simulink model "Droop_control_conditioning_untouched"  (R2024b)
settings: Solver=ode4  StartTime=0.0  StopTime=2  FixedStep=Ts  RelTol=1e-3
InitFcn:
  | %% Droop Control
  | m1=0.5e-5; % f-P droop gain
  | n1=5e-3;   % Q-V droop gain
  | fn=50;  % nominal frequency
  | Vn=325;  % nominal voltage
  | wc=2*pi*5;  % cut off frequency of low pass filter used in droop control
  | 
  | %% Voltage Controller
  | 
  | kpv=1;  % voltage controller proportional gain
  | kiv=189; % voltage controller integral gain
  | F=0.75;  % Feedforeward gain
  | Ilim1=40; % voltage controller limit
  | Ilim2=-40; % voltage controller limit
  | 
  | %% Current controller
  | 
  | kpi=10.47*2;  % current controller proportional gain
  | kii=4188.8*4; % current controller integral gain
  | Vlim1=500; % current controller limit
  | Vlim2=500; % current controller limit
  | 
  | %% System parameter
  | Lf=1.6e-3; % filter inductance
  | Cf=50e-6;  % filter capacitance
  | Rc=0.03;   % Coupling resistance
  | Lc=0.35e-3;% Coupling inducatnace
  | fs=10e3;    % switching frequency
  | Ts=10e-7;    % sample time
  | Vin=1000;   % DC voltage or input of inverter
  | Tsample=20*Ts;
  | ts=0.04; % black start time in step block used in Q-V droop controller and at PWM
  | 
  | %% Line parameters
  | R1=0.23; % line resistance
  | L1=3.1e-4;  %line inducatance
libraries: spsSeriesRLCBranchLib x9, slpidlib x8, spsThreePhaseSeriesRLCBranchLib x7, spsabctodq0Lib x6, spsGroundLib x5, spsThreePhaseVIMeasurementLib x5, spsDCVoltageSourceLib x2, spsPowerdq0InstantaneousLib x2, spsPWMGenerator2LevelLib x2, spsUniversalBridgeLib x2, spsdq0toabcLib x2, dspstat3 x1
(part 1 of 2)
settings Model: SimulationMode=accelerator  Creator=praki  LastModifiedBy=praki
settings DataIOCC: SaveFormat=StructureWithTime
settings RTWCC: GPUComputeCapability=3.5

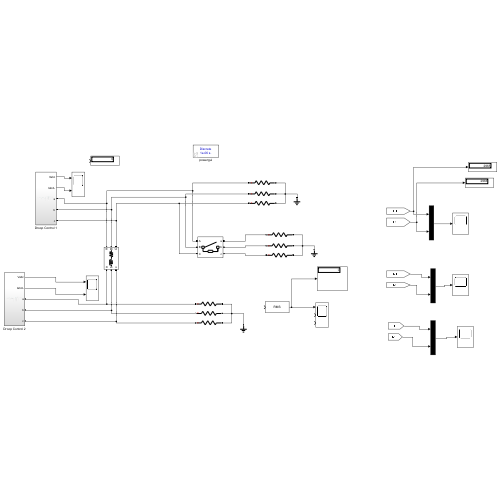
[thumbnail: Simulink's stored preview of the top-level diagram]
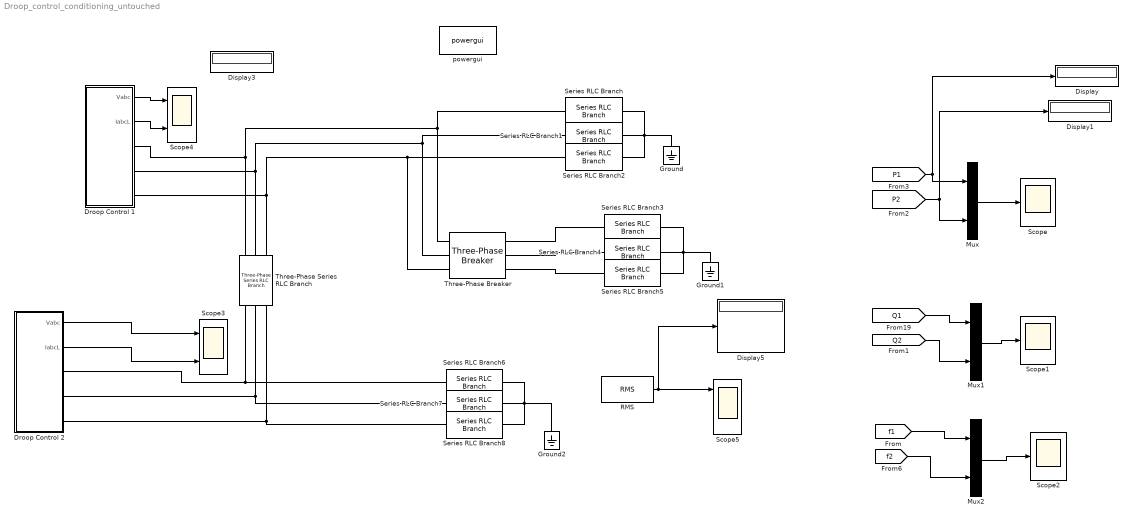
== system Droop_control_conditioning_untouched ==
  Display{,1,3,5} (4 alike) : Display
  Droop Control 1 : Subsystem
  Droop Control 2 : Subsystem
  Ground : spsGroundLib/Ground  LConnTagsString=a
  Ground1 : spsGroundLib/Ground  LConnTagsString=a
  Ground2 : spsGroundLib/Ground  LConnTagsString=a
  Mux : Mux  Inputs=2
  Mux1 : Mux  Inputs=2
  Mux2 : Mux  Inputs=2
  RMS : dspstat3/RMS  run=off  directionMode=Each column  dimension=1  InputProcessing=Columns as channels (frame based)  reset_popup=None
  Scope : Scope
  Scope1 : Scope
  Scope2 : Scope
  Scope3 : Scope  NumInputPorts=2
  Scope4 : Scope  NumInputPorts=2
  Scope5 : Scope  NumInputPorts=3
  Series RLC Branch : spsSeriesRLCBranchLib/Series RLC Branch  LConnTagsString=__new0  RConnTagsString=__new0  BranchType=R  Resistance=32  Inductance=1e-3  SetiL0=off  InitialCurrent=0  Capacitance=1e-6  Setx0=off  InitialVoltage=0  Measurements=None
  Series RLC Branch1 : spsSeriesRLCBranchLib/Series RLC Branch  LConnTagsString=__new0  RConnTagsString=__new0  BranchType=R  Resistance=32  Inductance=1e-3  SetiL0=off  InitialCurrent=0  Capacitance=1e-6  Setx0=off  InitialVoltage=0  Measurements=None
  Series RLC Branch2 : spsSeriesRLCBranchLib/Series RLC Branch  LConnTagsString=__new0  RConnTagsString=__new0  BranchType=R  Resistance=32  Inductance=1e-3  SetiL0=off  InitialCurrent=0  Capacitance=1e-6  Setx0=off  InitialVoltage=0  Measurements=None
  Series RLC Branch{3..8} (6 alike) : spsSeriesRLCBranchLib/Series RLC Branch  LConnTagsString=__new0  RConnTagsString=__new0  BranchType=R  Resistance=160  Inductance=1e-3  SetiL0=off  InitialCurrent=0  Capacitance=1e-6  Setx0=off  InitialVoltage=0  Measurements=None
  Three-Phase Series RLC Branch : spsThreePhaseSeriesRLCBranchLib/Three-Phase Series RLC Branch  LConnTagsString=A|B|C  RConnTagsString=A|B|C  BranchType=RL  Resistance=R1  Inductance=L1  Capacitance=1e-6  Measurements=None
  Three-Phase Breaker : spsThreePhaseBreakerLib/Three-Phase Breaker  InitialState=open  SwitchA=on  SwitchB=on  SwitchC=on  SwitchTimes=[1]  External=off  BreakerResistance=0.01  SnubberResistance=1e6  SnubberCapacitance=inf  Measurements=None
  powergui : sps_lib/powergui  Priority=1  SimulationMode=Discrete  SampleTime=Ts  frequency=60  Iterations=50  frequencyindice=0  Pbase=100e6  ErrMax=1e-4  UnitsV=kV  UnitsW=MW  buscounter=0  FunctionMessages=off  echomessages=off  EnableUseOfTLC=off  CurrentSourceSwitches=off  DisableSnubberDevices=off  DisableRonSwitches=off  DisableVfSwitches=off  DisplayEquations=off  AutomaticDiscreteSolvers=off  SolverType=Tustin/Backward Euler (TBE)  Interpol=off  ExternalGateDelay=off  methode=off  Ts=100  x0status=blocks  SPID=on  SwTol=0  HookPort=off  NonlinearTolerance=1e-4  nMaxIteration=100  ContinueOnMaxIteration=off  RestoreLinks=warning  ResistiveCurrentMeasurement=off  Frange=[0:2:500]  Ylog=off  Xlog=on  ShowGrid=off  save=off  variable=ZData  structure=0  ZoomFFT=off  StartTime=0.0  cycles=1  DisplayStyle=1  fundamental=60  FreqAxis=off  MaxFrequency=1000  frequencyindicesteady=1  RmsSteady=1  display=off
  wires:
  [P1] -> Display/1, Mux/1
  [f2] -> Mux2/2
  [P2] -> Display1/1, Mux/2
  Mux/1 -> Scope/1
  Mux2/1 -> Scope2/1
  [f1] -> Mux2/1
  Mux1/1 -> Scope1/1
  [Q1] -> Mux1/1
  [Q2] -> Mux1/2
  RMS/1 -> Display5/1, Scope5/1
  Droop Control 1/1(Vabc) -> Scope4/1
  Droop Control 1/2(IabcL) -> Scope4/2
  Droop Control 2/1(Vabc) -> Scope3/1
  Droop Control 2/2(IabcL) -> Scope3/2
  connections:
  Three-Phase Breaker/LConn2 -- Series RLC Branch1/LConn1 -- Three-Phase Series RLC Branch/LConn2 -- Droop Control 1/RConn2
  Three-Phase Breaker/LConn3 -- Series RLC Branch2/LConn1 -- Three-Phase Series RLC Branch/LConn3 -- Droop Control 1/RConn3
  Three-Phase Breaker/LConn1 -- Series RLC Branch/LConn1 -- Three-Phase Series RLC Branch/LConn1 -- Droop Control 1/RConn1
  Droop Control 2/RConn1 -- Three-Phase Series RLC Branch/RConn1 -- Series RLC Branch6/LConn1
  Droop Control 2/RConn2 -- Series RLC Branch7/LConn1 -- Three-Phase Series RLC Branch/RConn2
  Droop Control 2/RConn3 -- Series RLC Branch8/LConn1 -- Three-Phase Series RLC Branch/RConn3
  Series RLC Branch/RConn1 -- Series RLC Branch1/RConn1 -- Ground/LConn1 -- Series RLC Branch2/RConn1
  Series RLC Branch4/RConn1 -- Series RLC Branch5/RConn1 -- Ground1/LConn1 -- Series RLC Branch3/RConn1
  Series RLC Branch3/LConn1 -- Three-Phase Breaker/RConn1
  Three-Phase Breaker/RConn2 -- Series RLC Branch4/LConn1
  Three-Phase Breaker/RConn3 -- Series RLC Branch5/LConn1
  Series RLC Branch8/RConn1 -- Ground2/LConn1 -- Series RLC Branch7/RConn1 -- Series RLC Branch6/RConn1

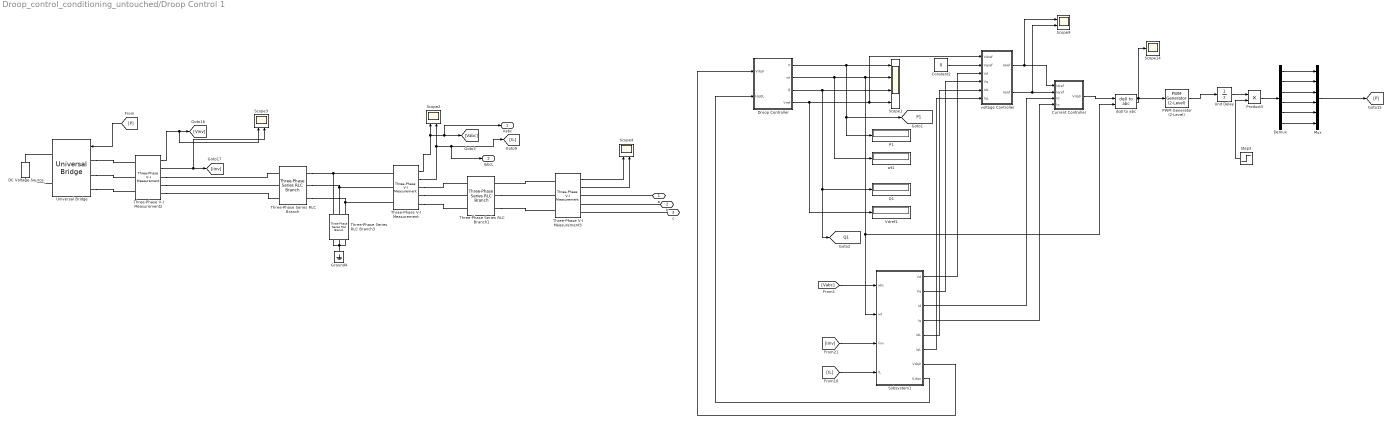
== system Droop_control_conditioning_untouched/Droop Control 1 ==
  Constant2 : Constant  Value=0
  Current Controller : Subsystem
  DC Voltage Source : spsDCVoltageSourceLib/DC Voltage Source  Amplitude=Vin  Measurements=None
  Demux : Demux  Outputs=6
  Droop Controller : Subsystem
  Ground4 : spsGroundLib/Ground  LConnTagsString=a
  Mux : Mux  Inputs=6
  P1 : Display
  PWM Generator (2-Level) : spsPWMGenerator2LevelLib/PWM Generator (2-Level)  ModulatorType=Three-phase bridge (6 pulses)  ModulatorMode=Unsynchronized  Fc=fs  Pc=90  nF=27  MinMax="[ -1  1 ]"  SamplingTechnique=Natural  ModulatingSignals=off  m=0.8  Freq=60  Phase=0  Ts=Ts  ShowCarrierOutport=off
  Product3 : Product  Inputs=**
  Q1 : Display
  Scope1 : Scope  NumInputPorts=4
  Scope14 : Scope
  Scope{2..4,9} (4 alike) : Scope  NumInputPorts=2
  Step3 : Step  Time=ts  SampleTime=0
  Subsystem1 : Subsystem
  Three-Phase Series RLC Branch : spsThreePhaseSeriesRLCBranchLib/Three-Phase Series RLC Branch  LConnTagsString=A|B|C  RConnTagsString=A|B|C  BranchType=RL  Resistance=0.2  Inductance=Lf  Capacitance=1e-6  Measurements=None
  Three-Phase Series RLC Branch1 : spsThreePhaseSeriesRLCBranchLib/Three-Phase Series RLC Branch  LConnTagsString=A|B|C  RConnTagsString=A|B|C  BranchType=RL  Resistance=Rc  Inductance=Lc  Capacitance=1e-6  Measurements=None
  Three-Phase Series RLC Branch3 : spsThreePhaseSeriesRLCBranchLib/Three-Phase Series RLC Branch  LConnTagsString=A|B|C  RConnTagsString=A|B|C  BranchType=C  Resistance=0.2  Inductance=50e-6  Capacitance=Cf  Measurements=None
  Three-Phase V-I Measurement : spsThreePhaseVIMeasurementLib/Three-Phase V-I Measurement  VoltageMeasurement=phase-to-ground  SetLabelV=off  LabelV=Vabc  Vpu=off  VpuLL=off  CurrentMeasurement=yes  SetLabelI=off  LabelI=Iload  Ipu=off  Pbase=100e6  Vbase=500e3  OutputType=Complex  PhasorSimulation=off  PSBequivalent=0
  Three-Phase V-I Measurement2 : spsThreePhaseVIMeasurementLib/Three-Phase V-I Measurement  VoltageMeasurement=phase-to-ground  SetLabelV=off  LabelV=Vabc  Vpu=off  VpuLL=off  CurrentMeasurement=yes  SetLabelI=off  LabelI=Iload  Ipu=off  Pbase=100e6  Vbase=500e3  OutputType=Complex  PhasorSimulation=off  PSBequivalent=0
  Three-Phase V-I Measurement3 : spsThreePhaseVIMeasurementLib/Three-Phase V-I Measurement  VoltageMeasurement=phase-to-ground  SetLabelV=off  LabelV=Vabc  Vpu=off  VpuLL=off  CurrentMeasurement=yes  SetLabelI=off  LabelI=Iload  Ipu=off  Pbase=100e6  Vbase=500e3  OutputType=Complex  PhasorSimulation=off  PSBequivalent=0
  Unit Delay : UnitDelay  SampleTime=Ts  HasFrameUpgradeWarning=on
  Universal Bridge : spsUniversalBridgeLib/Universal Bridge  Arms=3  SnubberResistance=1e5  SnubberCapacitance=inf  Device=IGBT / Diodes  Ron=1e-3  Lon=0  ForwardVoltages="[  0  0  ]"  ForwardVoltage=0  GTOparameters=[ 10e-6 , 20e-6 ]  IGBTparameters=[ 1e-6 , 2e-6 ]  Measurements=None  Measurements_2=None  converterType=Rectifier
  Vdref1 : Display
  dq0 to abc : spsdq0toabcLib/dq0 to abc  Alignment=90 degrees behind phase A axis
  voltage Controller : Subsystem
  wt1 : Display
  a : PMIOPort  Side=Right
  b : PMIOPort  Port=2  Side=Right
  c : PMIOPort  Port=3  Side=Right
  Vabc : Outport
  IabcL : Outport  Port=2
  tag scope: P1=global, Q1=global
  wires:
  Constant2/1 -> voltage Controller/2(Vqref)
  Three-Phase V-I Measurement/2 -> IabcL/1, [IL], Scope2/2
  Subsystem1/2(Vq) -> voltage Controller/4(Vq)
  Droop Controller/1(P) -> P1/1, [P1], Scope1/1
  Droop Controller/2(wt) -> wt1/1, Scope1/2, Subsystem1/2(wt), dq0 to abc/2
  Three-Phase V-I Measurement2/1 -> [Vinv], Scope3/1
  Three-Phase V-I Measurement/1 -> Vabc/1, [Vabc], Scope2/1
  [Iinv] -> Subsystem1/3(Iinv)
  Droop Controller/4(Vref) -> Vdref1/1, voltage Controller/1(Vdref), Scope1/4
  Droop Controller/3(Q) -> Q1/1, [Q1], Scope1/3
  dq0 to abc/1 -> PWM Generator (2-Level)/1, Scope14/1
  Subsystem1/3(Id) -> Current Controller/3(Id)
  [P] -> Universal Bridge/1
  Subsystem1/5(IdL) -> voltage Controller/5(IdL)
  Step3/1 -> Product3/2
  Subsystem1/8(ILdqo) -> Droop Controller/2(Idq0L)
  voltage Controller/1(Idref) -> Current Controller/1(Idref), Scope9/1
  Subsystem1/4(Iq) -> Current Controller/4(Iq)
  Unit Delay/1 -> Product3/1
  [Vabc] -> Subsystem1/1(abc)
  Subsystem1/6(IqL) -> voltage Controller/6(IqL)
  Subsystem1/7(Vdq0) -> Droop Controller/1(Vdq0)
  Three-Phase V-I Measurement2/2 -> Scope3/2, [Iinv]
  Current Controller/1(Vdq0) -> dq0 to abc/1
  Subsystem1/1(Vd) -> voltage Controller/3(Vd)
  [IL] -> Subsystem1/4(IL)
  voltage Controller/2(Iqref) -> Scope9/2, Current Controller/2(Iqref)
  Three-Phase V-I Measurement3/1 -> Scope4/1
  Three-Phase V-I Measurement3/2 -> Scope4/2
  PWM Generator (2-Level)/1 -> Unit Delay/1
  Demux/1 -> Mux/1
  Demux/2 -> Mux/2
  Demux/3 -> Mux/3
  Demux/4 -> Mux/4
  Demux/6 -> Mux/6
  Demux/5 -> Mux/5
  Product3/1 -> Demux/1
  Mux/1 -> [P]
  connections:
  DC Voltage Source/RConn1 -- Universal Bridge/RConn1
  Three-Phase V-I Measurement2/RConn1 -- Three-Phase Series RLC Branch/LConn1
  Three-Phase Series RLC Branch3/RConn2 -- Ground4/LConn1 -- Three-Phase Series RLC Branch3/RConn1 -- Three-Phase Series RLC Branch3/RConn3
  Three-Phase V-I Measurement2/RConn2 -- Three-Phase Series RLC Branch/LConn2
  Universal Bridge/LConn3 -- Three-Phase V-I Measurement2/LConn3
  Three-Phase Series RLC Branch/RConn3 -- Three-Phase V-I Measurement/LConn3 -- Three-Phase Series RLC Branch3/LConn3
  Three-Phase Series RLC Branch/RConn2 -- Three-Phase V-I Measurement/LConn2 -- Three-Phase Series RLC Branch3/LConn2
  Universal Bridge/LConn1 -- Three-Phase V-I Measurement2/LConn1
  Three-Phase Series RLC Branch/RConn1 -- Three-Phase V-I Measurement/LConn1 -- Three-Phase Series RLC Branch3/LConn1
  Universal Bridge/RConn2 -- DC Voltage Source/LConn1
  Three-Phase V-I Measurement2/RConn3 -- Three-Phase Series RLC Branch/LConn3
  Universal Bridge/LConn2 -- Three-Phase V-I Measurement2/LConn2
  Three-Phase V-I Measurement/RConn1 -- Three-Phase Series RLC Branch1/LConn1
  Three-Phase V-I Measurement/RConn2 -- Three-Phase Series RLC Branch1/LConn2
  Three-Phase V-I Measurement/RConn3 -- Three-Phase Series RLC Branch1/LConn3
  Three-Phase V-I Measurement3/LConn1 -- Three-Phase Series RLC Branch1/RConn1
  Three-Phase Series RLC Branch1/RConn2 -- Three-Phase V-I Measurement3/LConn2
  Three-Phase Series RLC Branch1/RConn3 -- Three-Phase V-I Measurement3/LConn3
  a/RConn1 -- Three-Phase V-I Measurement3/RConn1
  b/RConn1 -- Three-Phase V-I Measurement3/RConn2
  c/RConn1 -- Three-Phase V-I Measurement3/RConn3

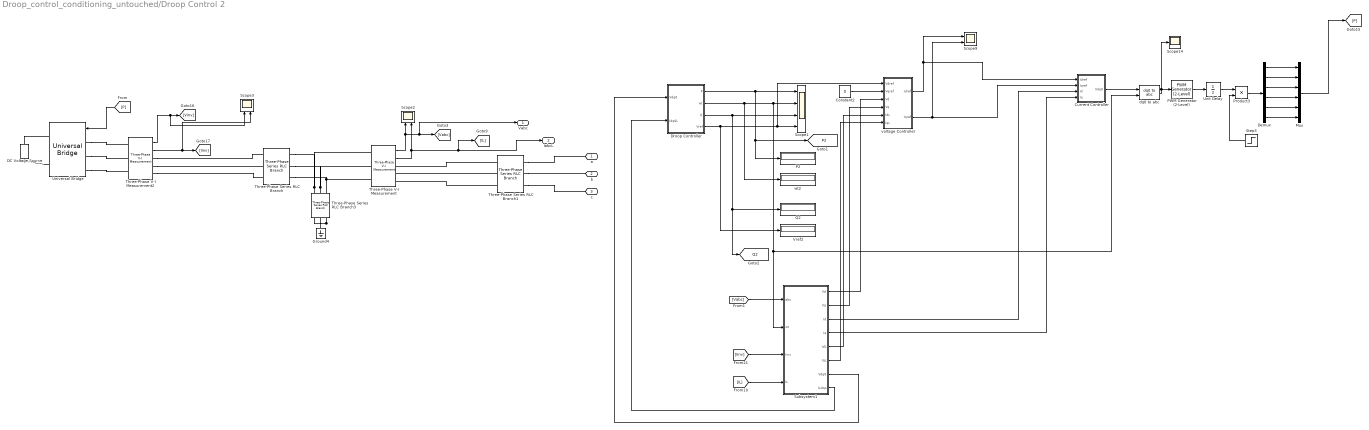
== system Droop_control_conditioning_untouched/Droop Control 2 ==
  Constant2 : Constant  Value=0
  Current Controller : Subsystem
  DC Voltage Source : spsDCVoltageSourceLib/DC Voltage Source  Amplitude=Vin  Measurements=None
  Demux : Demux  Outputs=6
  Droop Controller : Subsystem
  Ground4 : spsGroundLib/Ground  LConnTagsString=a
  Mux : Mux  Inputs=6
  P2 : Display
  PWM Generator (2-Level) : spsPWMGenerator2LevelLib/PWM Generator (2-Level)  ModulatorType=Three-phase bridge (6 pulses)  ModulatorMode=Unsynchronized  Fc=fs  Pc=90  nF=27  MinMax="[ -1  1 ]"  SamplingTechnique=Natural  ModulatingSignals=off  m=0.8  Freq=60  Phase=0  Ts=Ts  ShowCarrierOutport=off
  Product3 : Product  Inputs=**
  Q2 : Display
  Scope1 : Scope  NumInputPorts=4
  Scope14 : Scope
  Scope2 : Scope  NumInputPorts=2
  Scope3 : Scope  NumInputPorts=2
  Scope9 : Scope  NumInputPorts=2
  Step3 : Step  Time=ts  SampleTime=0
  Subsystem1 : Subsystem
  Three-Phase Series RLC Branch : spsThreePhaseSeriesRLCBranchLib/Three-Phase Series RLC Branch  LConnTagsString=A|B|C  RConnTagsString=A|B|C  BranchType=RL  Resistance=0.2  Inductance=Lf  Capacitance=1e-6  Measurements=None
  Three-Phase Series RLC Branch1 : spsThreePhaseSeriesRLCBranchLib/Three-Phase Series RLC Branch  LConnTagsString=A|B|C  RConnTagsString=A|B|C  BranchType=RL  Resistance=Rc  Inductance=Lc  Capacitance=1e-6  Measurements=None
  Three-Phase Series RLC Branch3 : spsThreePhaseSeriesRLCBranchLib/Three-Phase Series RLC Branch  LConnTagsString=A|B|C  RConnTagsString=A|B|C  BranchType=C  Resistance=0.2  Inductance=50e-6  Capacitance=Cf  Measurements=None
  Three-Phase V-I Measurement : spsThreePhaseVIMeasurementLib/Three-Phase V-I Measurement  VoltageMeasurement=phase-to-ground  SetLabelV=off  LabelV=Vabc  Vpu=off  VpuLL=off  CurrentMeasurement=yes  SetLabelI=off  LabelI=Iload  Ipu=off  Pbase=100e6  Vbase=500e3  OutputType=Complex  PhasorSimulation=off  PSBequivalent=0
  Three-Phase V-I Measurement2 : spsThreePhaseVIMeasurementLib/Three-Phase V-I Measurement  VoltageMeasurement=phase-to-ground  SetLabelV=off  LabelV=Vabc  Vpu=off  VpuLL=off  CurrentMeasurement=yes  SetLabelI=off  LabelI=Iload  Ipu=off  Pbase=100e6  Vbase=500e3  OutputType=Complex  PhasorSimulation=off  PSBequivalent=0
  Unit Delay : UnitDelay  SampleTime=Ts  HasFrameUpgradeWarning=on
  Universal Bridge : spsUniversalBridgeLib/Universal Bridge  Arms=3  SnubberResistance=1e5  SnubberCapacitance=inf  Device=IGBT / Diodes  Ron=1e-3  Lon=0  ForwardVoltages="[  0  0  ]"  ForwardVoltage=0  GTOparameters=[ 10e-6 , 20e-6 ]  IGBTparameters=[ 1e-6 , 2e-6 ]  Measurements=None  Measurements_2=None  converterType=Rectifier
  Vref2 : Display
  dq0 to abc : spsdq0toabcLib/dq0 to abc  Alignment=90 degrees behind phase A axis
  voltage Controller : Subsystem
  wt2 : Display
  a : PMIOPort  Side=Right
  b : PMIOPort  Port=2  Side=Right
  c : PMIOPort  Port=3  Side=Right
  Vabc : Outport
  IabcL : Outport  Port=2
  tag scope: P2=global, Q2=global
  wires:
  [IL] -> Subsystem1/4(IL)
  Subsystem1/1(Vd) -> voltage Controller/3(Vd)
  Current Controller/1(Vdq0) -> dq0 to abc/1
  Three-Phase V-I Measurement2/2 -> [Iinv], Scope3/2
  Subsystem1/7(Vdq0) -> Droop Controller/1(Vdq0)
  Subsystem1/6(IqL) -> voltage Controller/6(IqL)
  [Vabc] -> Subsystem1/1(abc)
  Unit Delay/1 -> Product3/1
  Subsystem1/4(Iq) -> Current Controller/4(Iq)
  voltage Controller/1(Idref) -> Current Controller/1(Idref), Scope9/1
  Subsystem1/8(ILdqo) -> Droop Controller/2(Idq0L)
  Step3/1 -> Product3/2
  Subsystem1/5(IdL) -> voltage Controller/5(IdL)
  [P] -> Universal Bridge/1
  Subsystem1/3(Id) -> Current Controller/3(Id)
  dq0 to abc/1 -> Scope14/1, PWM Generator (2-Level)/1
  Droop Controller/3(Q) -> Scope1/3, [Q2], Q2/1
  Droop Controller/4(Vref) -> Scope1/4, voltage Controller/1(Vdref), Vref2/1
  [Iinv] -> Subsystem1/3(Iinv)
  Three-Phase V-I Measurement/1 -> Scope2/1, Vabc/1, [Vabc]
  Three-Phase V-I Measurement2/1 -> Scope3/1, [Vinv]
  Droop Controller/2(wt) -> dq0 to abc/2, Subsystem1/2(wt), Scope1/2, wt2/1
  Droop Controller/1(P) -> Scope1/1, [P2], P2/1
  Subsystem1/2(Vq) -> voltage Controller/4(Vq)
  Three-Phase V-I Measurement/2 -> Scope2/2, IabcL/1, [IL]
  Constant2/1 -> voltage Controller/2(Vqref)
  voltage Controller/2(Iqref) -> Scope9/2, Current Controller/2(Iqref)
  PWM Generator (2-Level)/1 -> Unit Delay/1
  Mux/1 -> [P]
  Demux/5 -> Mux/5
  Product3/1 -> Demux/1
  Demux/3 -> Mux/3
  Demux/2 -> Mux/2
  Demux/1 -> Mux/1
  Demux/4 -> Mux/4
  Demux/6 -> Mux/6
  connections:
  Universal Bridge/LConn2 -- Three-Phase V-I Measurement2/LConn2
  Three-Phase V-I Measurement2/RConn3 -- Three-Phase Series RLC Branch/LConn3
  Universal Bridge/RConn2 -- DC Voltage Source/LConn1
  Three-Phase Series RLC Branch3/LConn1 -- Three-Phase Series RLC Branch/RConn1 -- Three-Phase V-I Measurement/LConn1
  Universal Bridge/LConn1 -- Three-Phase V-I Measurement2/LConn1
  Three-Phase Series RLC Branch3/LConn2 -- Three-Phase Series RLC Branch/RConn2 -- Three-Phase V-I Measurement/LConn2
  Three-Phase Series RLC Branch/RConn3 -- Three-Phase V-I Measurement/LConn3 -- Three-Phase Series RLC Branch3/LConn3
  Universal Bridge/LConn3 -- Three-Phase V-I Measurement2/LConn3
  Three-Phase V-I Measurement2/RConn2 -- Three-Phase Series RLC Branch/LConn2
  Three-Phase Series RLC Branch3/RConn3 -- Three-Phase Series RLC Branch3/RConn1 -- Three-Phase Series RLC Branch3/RConn2 -- Ground4/LConn1
  Three-Phase V-I Measurement2/RConn1 -- Three-Phase Series RLC Branch/LConn1
  DC Voltage Source/RConn1 -- Universal Bridge/RConn1
  Three-Phase Series RLC Branch1/LConn1 -- Three-Phase V-I Measurement/RConn1
  Three-Phase Series RLC Branch1/LConn2 -- Three-Phase V-I Measurement/RConn2
  Three-Phase Series RLC Branch1/LConn3 -- Three-Phase V-I Measurement/RConn3
  Three-Phase Series RLC Branch1/RConn1 -- a/RConn1
  Three-Phase Series RLC Branch1/RConn2 -- b/RConn1
  Three-Phase Series RLC Branch1/RConn3 -- c/RConn1

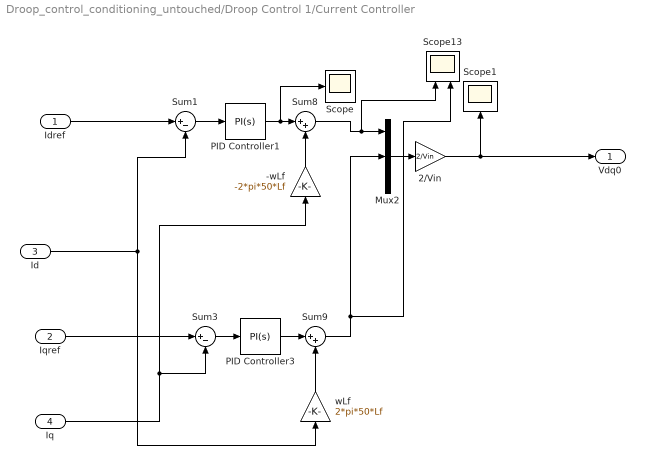
== system Droop_control_conditioning_untouched/Droop Control 1/Current Controller ==
  Idref : Inport
  Iqref : Inport  Port=2
  Id : Inport  Port=3
  Iq : Inport  Port=4
  -wLf : Gain  Gain=-2*pi*50*Lf
  2/Vin : Gain  Gain=2/Vin
  Mux2 : Mux  Inputs=3
  PID Controller1 : slpidlib/PID Controller  Controller=PI  Form=Parallel  TimeDomain=Continuous-time  UseExternalTs=off  SampleTime=Tsample  IntegratorMethod=Forward Euler  FilterMethod=Forward Euler  ControllerParametersSource=internal  P=kpi  I=kii  UseKiTs=off  D=0  UseExternalDerivativeSource=off  N=100  UseFilter=on  TunerSelectOption=Transfer Function Based (PID Tuner App)  InitialConditionSource=internal  InitialConditionForIntegrator=0  InitialConditionForFilter=0  DifferentiatorICPrevScaledInput=0  ExternalReset=none  TrackingMode=off  Kt=1  LimitOutput=off  SatLimitsSource=internal  UpperSaturationLimit=Vlim1  LowerSaturationLimit=Vlim2  LinearizeAsGain=on  AntiWindupMode=none  Kb=1  LimitIntegrator=off  UpperIntegratorSaturationLimit=inf  LowerIntegratorSaturationLimit=-inf  POutMin=[]  POutMax=[]  IOutMin=[]  IOutMax=[]  DOutMin=[]  DOutMax=[]  NOutMin=[]  NOutMax=[]  SumOutMin=[]  SumOutMax=[]  SaturationOutMin=[]  SaturationOutMax=[]  PParamMin=[]  PParamMax=[]  IParamMin=[]  IParamMax=[]  DParamMin=[]  DParamMax=[]  NParamMin=[]  NParamMax=[]  KbParamMin=[]  KbParamMax=[]  KtParamMin=[]  KtParamMax=[]  KbOutMin=[]  KbOutMax=[]  KtOutMin=[]  KtOutMax=[]  IntegratorOutMin=[]  IntegratorOutMax=[]  FilterOutMin=[]  FilterOutMax=[]  SumI1OutMin=[]  SumI1OutMax=[]  SumI2OutMin=[]  SumI2OutMax=[]  SumI3OutMin=[]  SumI3OutMax=[]  SumI4OutMin=[]  SumI4OutMax=[]  SumDOutMin=[]  SumDOutMax=[]  DifferentiatorOutMin=[]  DifferentiatorOutMax=[]  FilterDiffOutCoefMin=[]  FilterDiffOutCoefMax=[]  ReciprocalOutMin=[]  ReciprocalOutMax=[]  SumDenOutMin=[]  SumDenOutMax=[]  SumNumOutMin=[]  SumNumOutMax=[]  DivideOutMin=[]  DivideOutMax=[]  UdiffTsProdOutMin=[]  UdiffTsProdOutMax=[]  NTsProdOutMin=[]  NTsProdOutMax=[]  UintegralTsProdOutMin=[]  UintegralTsProdOutMax=[]  UngainTsProdOutMin=[]  UngainTsProdOutMax=[]  ClampingZeroOutDataTypeStr=Inherit: Inherit via back propagation  ClampingZeroOutMin=[]  ClampingZeroOutMax=[]  FilterDenConstantOutDataTypeStr=Inherit: Inherit via back propagation  FilterDenConstantOutMin=[]  FilterDenConstantOutMax=[]  PCopyOutDataTypeStr=Inherit: Inherit via back propagation  PCopyOutMin=[]  PCopyOutMax=[]  NCopyOutDataTypeStr=Inherit: Inherit via back propagation  NCopyOutMin=[]  NCopyOutMax=[]  IntegratorContinuousStateAttributes=''  IntegratorStateMustResolveToSignalObject=off  IntegratorRTWStateStorageClass=Auto  FilterContinuousStateAttributes=''  FilterStateMustResolveToSignalObject=off  FilterRTWStateStorageClass=Auto  ParallelPVariant=InternalParameters  IdealPVariant=Disabled  IVariant=InternalParameters  DVariant=Disabled  IntegratorVariant=Continuous  SatVariant=Disabled  AWVariant=Passthrough  PCopyVariant=Disabled  TRVariant=Disabled  FdbkBlocksVariant=Forward  IdealPFdbkVariant=Disabled  SatFdbkVariant=Disabled  DerivativeFilterVariant=Disabled  NVariant=Disabled  NCopyVariant=Disabled_SignalSpec  FilterICVariant=Disabled  IntegratorICVariant=InternalICs  ExternalResetVariant=Disabled  TRSumVariant=Passthrough  SumFdbkVariant=Disabled  SumVariant=Sum_PI  TsampFilterVariant=InternalTs  TsampNgainVariant=Passthrough  TsampIntegralVariant=Disabled_SignalSpec  ExternalSaturationOutDataTypeStr=Inherit: Same as second input  DerivativeSourceVariant=Disabled  PreIntVariant=InternalPreInt
  PID Controller3 : slpidlib/PID Controller  Controller=PI  Form=Parallel  TimeDomain=Continuous-time  UseExternalTs=off  SampleTime=Tsample  IntegratorMethod=Forward Euler  FilterMethod=Forward Euler  ControllerParametersSource=internal  P=kpi  I=kii  UseKiTs=off  D=0  UseExternalDerivativeSource=off  N=100  UseFilter=on  TunerSelectOption=Transfer Function Based (PID Tuner App)  InitialConditionSource=internal  InitialConditionForIntegrator=0  InitialConditionForFilter=0  DifferentiatorICPrevScaledInput=0  ExternalReset=none  TrackingMode=off  Kt=1  LimitOutput=off  SatLimitsSource=internal  UpperSaturationLimit=Vlim1  LowerSaturationLimit=Vlim2  LinearizeAsGain=on  AntiWindupMode=none  Kb=1  LimitIntegrator=off  UpperIntegratorSaturationLimit=inf  LowerIntegratorSaturationLimit=-inf  POutMin=[]  POutMax=[]  IOutMin=[]  IOutMax=[]  DOutMin=[]  DOutMax=[]  NOutMin=[]  NOutMax=[]  SumOutMin=[]  SumOutMax=[]  SaturationOutMin=[]  SaturationOutMax=[]  PParamMin=[]  PParamMax=[]  IParamMin=[]  IParamMax=[]  DParamMin=[]  DParamMax=[]  NParamMin=[]  NParamMax=[]  KbParamMin=[]  KbParamMax=[]  KtParamMin=[]  KtParamMax=[]  KbOutMin=[]  KbOutMax=[]  KtOutMin=[]  KtOutMax=[]  IntegratorOutMin=[]  IntegratorOutMax=[]  FilterOutMin=[]  FilterOutMax=[]  SumI1OutMin=[]  SumI1OutMax=[]  SumI2OutMin=[]  SumI2OutMax=[]  SumI3OutMin=[]  SumI3OutMax=[]  SumI4OutMin=[]  SumI4OutMax=[]  SumDOutMin=[]  SumDOutMax=[]  DifferentiatorOutMin=[]  DifferentiatorOutMax=[]  FilterDiffOutCoefMin=[]  FilterDiffOutCoefMax=[]  ReciprocalOutMin=[]  ReciprocalOutMax=[]  SumDenOutMin=[]  SumDenOutMax=[]  SumNumOutMin=[]  SumNumOutMax=[]  DivideOutMin=[]  DivideOutMax=[]  UdiffTsProdOutMin=[]  UdiffTsProdOutMax=[]  NTsProdOutMin=[]  NTsProdOutMax=[]  UintegralTsProdOutMin=[]  UintegralTsProdOutMax=[]  UngainTsProdOutMin=[]  UngainTsProdOutMax=[]  ClampingZeroOutDataTypeStr=Inherit: Inherit via back propagation  ClampingZeroOutMin=[]  ClampingZeroOutMax=[]  FilterDenConstantOutDataTypeStr=Inherit: Inherit via back propagation  FilterDenConstantOutMin=[]  FilterDenConstantOutMax=[]  PCopyOutDataTypeStr=Inherit: Inherit via back propagation  PCopyOutMin=[]  PCopyOutMax=[]  NCopyOutDataTypeStr=Inherit: Inherit via back propagation  NCopyOutMin=[]  NCopyOutMax=[]  IntegratorContinuousStateAttributes=''  IntegratorStateMustResolveToSignalObject=off  IntegratorRTWStateStorageClass=Auto  FilterContinuousStateAttributes=''  FilterStateMustResolveToSignalObject=off  FilterRTWStateStorageClass=Auto  ParallelPVariant=InternalParameters  IdealPVariant=Disabled  IVariant=InternalParameters  DVariant=Disabled  IntegratorVariant=Continuous  SatVariant=Disabled  AWVariant=Passthrough  PCopyVariant=Disabled  TRVariant=Disabled  FdbkBlocksVariant=Forward  IdealPFdbkVariant=Disabled  SatFdbkVariant=Disabled  DerivativeFilterVariant=Disabled  NVariant=Disabled  NCopyVariant=Disabled_SignalSpec  FilterICVariant=Disabled  IntegratorICVariant=InternalICs  ExternalResetVariant=Disabled  TRSumVariant=Passthrough  SumFdbkVariant=Disabled  SumVariant=Sum_PI  TsampFilterVariant=InternalTs  TsampNgainVariant=Passthrough  TsampIntegralVariant=Disabled_SignalSpec  ExternalSaturationOutDataTypeStr=Inherit: Same as second input  DerivativeSourceVariant=Disabled  PreIntVariant=InternalPreInt
  Scope : Scope
  Scope1 : Scope
  Scope13 : Scope  NumInputPorts=2
  Sum1 : Sum  Inputs=|+-
  Sum3 : Sum  Inputs=|+-
  Sum8 : Sum  Inputs=|++
  Sum9 : Sum  Inputs=|++
  wLf : Gain  Gain=2*pi*50*Lf
  Vdq0 : Outport
  wires:
  Sum9/1 -> Scope13/2, Mux2/2
  wLf/1 -> Sum9/2
  2/Vin/1 -> Vdq0/1, Scope1/1
  Id/1 -> Sum1/2, wLf/1
  Iq/1 -> -wLf/1, Sum3/2
  Sum1/1 -> PID Controller1/1
  PID Controller3/1 -> Sum9/1
  Sum8/1 -> Scope13/1, Mux2/1
  Sum3/1 -> PID Controller3/1
  PID Controller1/1 -> Scope/1, Sum8/1
  Mux2/1 -> 2/Vin/1
  Idref/1 -> Sum1/1
  -wLf/1 -> Sum8/2
  Iqref/1 -> Sum3/1

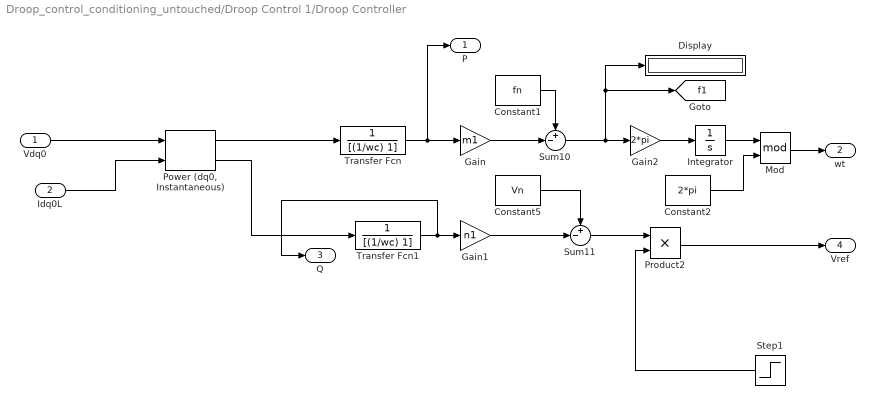
== system Droop_control_conditioning_untouched/Droop Control 1/Droop Controller ==
  Vdq0 : Inport
  Idq0L : Inport  Port=2
  Constant1 : Constant  Value=fn
  Constant2 : Constant  Value=2*pi
  Constant5 : Constant  Value=Vn
  Display : Display
  Gain : Gain  Gain=m1
  Gain1 : Gain  Gain=n1
  Gain2 : Gain  Gain=2*pi
  Integrator : Integrator
  Mod : Math  Operator=mod
  "Power (dq0, Instantaneous)" : spsPowerdq0InstantaneousLib/Power (dq0, Instantaneous)
      settings: LibrarySourceBlock=|
      | sps_lib/Sensors and Measurements/Power
      | (dq0, Instantaneous)
  Product2 : Product  Inputs=**
  Step1 : Step  Time=ts  SampleTime=0
  Sum10 : Sum  Inputs=+-|
  Sum11 : Sum  Inputs=+-|
  Transfer Fcn : TransferFcn  Numerator=[0 1]  Denominator=[(1/wc) 1]
  Transfer Fcn1 : TransferFcn  Numerator=[0 1]  Denominator=[(1/wc) 1]
  P : Outport
  wt : Outport  Port=2
  Q : Outport  Port=3
  Vref : Outport  Port=4
  tag scope: f1=global
  wires:
  "Power (dq0, Instantaneous)"/2 -> Transfer Fcn1/1
  "Power (dq0, Instantaneous)"/1 -> Transfer Fcn/1
  Constant1/1 -> Sum10/1
  Constant5/1 -> Sum11/1
  Gain1/1 -> Sum11/2
  Gain/1 -> Sum10/2
  Transfer Fcn/1 -> P/1, Gain/1
  Transfer Fcn1/1 -> Q/1, Gain1/1
  Integrator/1 -> Mod/1
  Mod/1 -> wt/1
  Constant2/1 -> Mod/2
  Vdq0/1 -> "Power (dq0, Instantaneous)"/1
  Idq0L/1 -> "Power (dq0, Instantaneous)"/2
  Gain2/1 -> Integrator/1
  Sum10/1 -> Gain2/1, [f1], Display/1
  Step1/1 -> Product2/2
  Product2/1 -> Vref/1
  Sum11/1 -> Product2/1

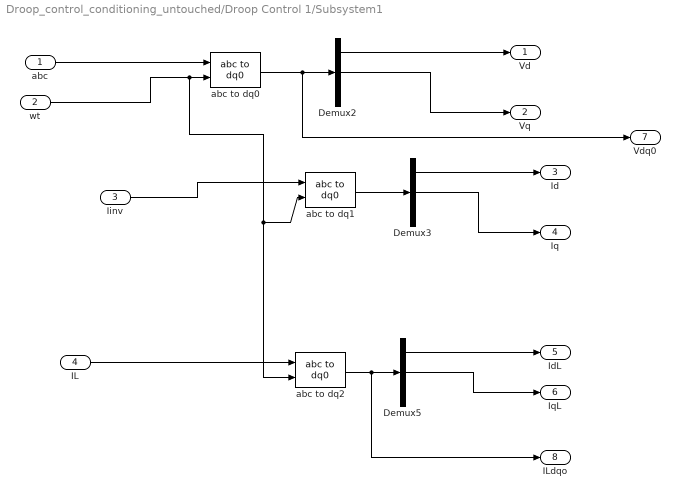
== system Droop_control_conditioning_untouched/Droop Control 1/Subsystem1 ==
  abc : Inport
  wt : Inport  Port=2
  Iinv : Inport  Port=3
  IL : Inport  Port=4
  Demux2 : Demux  Outputs=3
  Demux3 : Demux  Outputs=3
  Demux5 : Demux  Outputs=3
  abc to dq0 : spsabctodq0Lib/abc to dq0  Alignment=90 degrees behind phase A axis
  abc to dq1 : spsabctodq0Lib/abc to dq0  Alignment=90 degrees behind phase A axis
  abc to dq2 : spsabctodq0Lib/abc to dq0  Alignment=90 degrees behind phase A axis
  Vd : Outport
  Vq : Outport  Port=2
  Id : Outport  Port=3
  Iq : Outport  Port=4
  IdL : Outport  Port=5
  IqL : Outport  Port=6
  Vdq0 : Outport  Port=7
  ILdqo : Outport  Port=8
  wires:
  abc to dq0/1 -> Vdq0/1, Demux2/1
  abc to dq2/1 -> ILdqo/1, Demux5/1
  abc to dq1/1 -> Demux3/1
  wt/1 -> abc to dq2/2, abc to dq1/2, abc to dq0/2
  Demux2/2 -> Vq/1
  Iinv/1 -> abc to dq1/1
  Demux3/1 -> Id/1
  Demux2/1 -> Vd/1
  Demux5/1 -> IdL/1
  Demux5/2 -> IqL/1
  abc/1 -> abc to dq0/1
  Demux3/2 -> Iq/1
  IL/1 -> abc to dq2/1

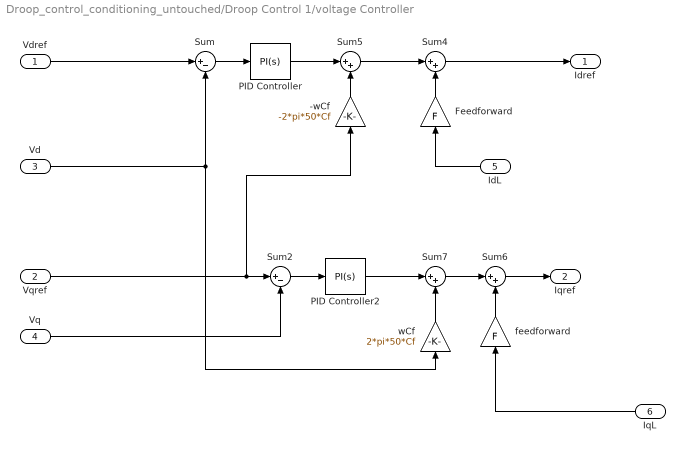
== system Droop_control_conditioning_untouched/Droop Control 1/voltage Controller ==
  Vdref : Inport
  Vqref : Inport  Port=2
  Vd : Inport  Port=3
  Vq : Inport  Port=4
  IdL : Inport  Port=5
  IqL : Inport  Port=6
  -wCf : Gain  Gain=-2*pi*50*Cf
  Feedforward : Gain  Gain=F
  PID Controller : slpidlib/PID Controller  Controller=PI  Form=Parallel  TimeDomain=Continuous-time  UseExternalTs=off  SampleTime=Tsample  IntegratorMethod=Forward Euler  FilterMethod=Forward Euler  ControllerParametersSource=internal  P=kpv  I=kiv  UseKiTs=off  D=0  UseExternalDerivativeSource=off  N=100  UseFilter=on  TunerSelectOption=Transfer Function Based (PID Tuner App)  InitialConditionSource=internal  InitialConditionForIntegrator=0  InitialConditionForFilter=0  DifferentiatorICPrevScaledInput=0  ExternalReset=none  TrackingMode=off  Kt=1  LimitOutput=off  SatLimitsSource=internal  UpperSaturationLimit=Ilim1  LowerSaturationLimit=Ilim2  LinearizeAsGain=off  AntiWindupMode=none  Kb=1  LimitIntegrator=off  UpperIntegratorSaturationLimit=inf  LowerIntegratorSaturationLimit=-inf  POutMin=[]  POutMax=[]  IOutMin=[]  IOutMax=[]  DOutMin=[]  DOutMax=[]  NOutMin=[]  NOutMax=[]  SumOutMin=[]  SumOutMax=[]  SaturationOutMin=[]  SaturationOutMax=[]  PParamMin=[]  PParamMax=[]  IParamMin=[]  IParamMax=[]  DParamMin=[]  DParamMax=[]  NParamMin=[]  NParamMax=[]  KbParamMin=[]  KbParamMax=[]  KtParamMin=[]  KtParamMax=[]  KbOutMin=[]  KbOutMax=[]  KtOutMin=[]  KtOutMax=[]  IntegratorOutMin=[]  IntegratorOutMax=[]  FilterOutMin=[]  FilterOutMax=[]  SumI1OutMin=[]  SumI1OutMax=[]  SumI2OutMin=[]  SumI2OutMax=[]  SumI3OutMin=[]  SumI3OutMax=[]  SumI4OutMin=[]  SumI4OutMax=[]  SumDOutMin=[]  SumDOutMax=[]  DifferentiatorOutMin=[]  DifferentiatorOutMax=[]  FilterDiffOutCoefMin=[]  FilterDiffOutCoefMax=[]  ReciprocalOutMin=[]  ReciprocalOutMax=[]  SumDenOutMin=[]  SumDenOutMax=[]  SumNumOutMin=[]  SumNumOutMax=[]  DivideOutMin=[]  DivideOutMax=[]  UdiffTsProdOutMin=[]  UdiffTsProdOutMax=[]  NTsProdOutMin=[]  NTsProdOutMax=[]  UintegralTsProdOutMin=[]  UintegralTsProdOutMax=[]  UngainTsProdOutMin=[]  UngainTsProdOutMax=[]  ClampingZeroOutDataTypeStr=Inherit: Inherit via back propagation  ClampingZeroOutMin=[]  ClampingZeroOutMax=[]  FilterDenConstantOutDataTypeStr=Inherit: Inherit via back propagation  FilterDenConstantOutMin=[]  FilterDenConstantOutMax=[]  PCopyOutDataTypeStr=Inherit: Inherit via back propagation  PCopyOutMin=[]  PCopyOutMax=[]  NCopyOutDataTypeStr=Inherit: Inherit via back propagation  NCopyOutMin=[]  NCopyOutMax=[]  IntegratorContinuousStateAttributes=''  IntegratorStateMustResolveToSignalObject=off  IntegratorRTWStateStorageClass=Auto  FilterContinuousStateAttributes=''  FilterStateMustResolveToSignalObject=off  FilterRTWStateStorageClass=Auto  ParallelPVariant=InternalParameters  IdealPVariant=Disabled  IVariant=InternalParameters  DVariant=Disabled  IntegratorVariant=Continuous  SatVariant=Disabled  AWVariant=Passthrough  PCopyVariant=Disabled  TRVariant=Disabled  FdbkBlocksVariant=Forward  IdealPFdbkVariant=Disabled  SatFdbkVariant=Disabled  DerivativeFilterVariant=Disabled  NVariant=Disabled  NCopyVariant=Disabled_SignalSpec  FilterICVariant=Disabled  IntegratorICVariant=InternalICs  ExternalResetVariant=Disabled  TRSumVariant=Passthrough  SumFdbkVariant=Disabled  SumVariant=Sum_PI  TsampFilterVariant=InternalTs  TsampNgainVariant=Passthrough  TsampIntegralVariant=Disabled_SignalSpec  ExternalSaturationOutDataTypeStr=Inherit: Same as second input  DerivativeSourceVariant=Disabled  PreIntVariant=InternalPreInt
  PID Controller2 : slpidlib/PID Controller  Controller=PI  Form=Parallel  TimeDomain=Continuous-time  UseExternalTs=off  SampleTime=Tsample  IntegratorMethod=Forward Euler  FilterMethod=Forward Euler  ControllerParametersSource=internal  P=kpv  I=kiv  UseKiTs=off  D=0  UseExternalDerivativeSource=off  N=100  UseFilter=on  TunerSelectOption=Transfer Function Based (PID Tuner App)  InitialConditionSource=internal  InitialConditionForIntegrator=0  InitialConditionForFilter=0  DifferentiatorICPrevScaledInput=0  ExternalReset=none  TrackingMode=off  Kt=1  LimitOutput=off  SatLimitsSource=internal  UpperSaturationLimit=Ilim1  LowerSaturationLimit=Ilim2  LinearizeAsGain=off  AntiWindupMode=none  Kb=1  LimitIntegrator=off  UpperIntegratorSaturationLimit=inf  LowerIntegratorSaturationLimit=-inf  POutMin=[]  POutMax=[]  IOutMin=[]  IOutMax=[]  DOutMin=[]  DOutMax=[]  NOutMin=[]  NOutMax=[]  SumOutMin=[]  SumOutMax=[]  SaturationOutMin=[]  SaturationOutMax=[]  PParamMin=[]  PParamMax=[]  IParamMin=[]  IParamMax=[]  DParamMin=[]  DParamMax=[]  NParamMin=[]  NParamMax=[]  KbParamMin=[]  KbParamMax=[]  KtParamMin=[]  KtParamMax=[]  KbOutMin=[]  KbOutMax=[]  KtOutMin=[]  KtOutMax=[]  IntegratorOutMin=[]  IntegratorOutMax=[]  FilterOutMin=[]  FilterOutMax=[]  SumI1OutMin=[]  SumI1OutMax=[]  SumI2OutMin=[]  SumI2OutMax=[]  SumI3OutMin=[]  SumI3OutMax=[]  SumI4OutMin=[]  SumI4OutMax=[]  SumDOutMin=[]  SumDOutMax=[]  DifferentiatorOutMin=[]  DifferentiatorOutMax=[]  FilterDiffOutCoefMin=[]  FilterDiffOutCoefMax=[]  ReciprocalOutMin=[]  ReciprocalOutMax=[]  SumDenOutMin=[]  SumDenOutMax=[]  SumNumOutMin=[]  SumNumOutMax=[]  DivideOutMin=[]  DivideOutMax=[]  UdiffTsProdOutMin=[]  UdiffTsProdOutMax=[]  NTsProdOutMin=[]  NTsProdOutMax=[]  UintegralTsProdOutMin=[]  UintegralTsProdOutMax=[]  UngainTsProdOutMin=[]  UngainTsProdOutMax=[]  ClampingZeroOutDataTypeStr=Inherit: Inherit via back propagation  ClampingZeroOutMin=[]  ClampingZeroOutMax=[]  FilterDenConstantOutDataTypeStr=Inherit: Inherit via back propagation  FilterDenConstantOutMin=[]  FilterDenConstantOutMax=[]  PCopyOutDataTypeStr=Inherit: Inherit via back propagation  PCopyOutMin=[]  PCopyOutMax=[]  NCopyOutDataTypeStr=Inherit: Inherit via back propagation  NCopyOutMin=[]  NCopyOutMax=[]  IntegratorContinuousStateAttributes=''  IntegratorStateMustResolveToSignalObject=off  IntegratorRTWStateStorageClass=Auto  FilterContinuousStateAttributes=''  FilterStateMustResolveToSignalObject=off  FilterRTWStateStorageClass=Auto  ParallelPVariant=InternalParameters  IdealPVariant=Disabled  IVariant=InternalParameters  DVariant=Disabled  IntegratorVariant=Continuous  SatVariant=Disabled  AWVariant=Passthrough  PCopyVariant=Disabled  TRVariant=Disabled  FdbkBlocksVariant=Forward  IdealPFdbkVariant=Disabled  SatFdbkVariant=Disabled  DerivativeFilterVariant=Disabled  NVariant=Disabled  NCopyVariant=Disabled_SignalSpec  FilterICVariant=Disabled  IntegratorICVariant=InternalICs  ExternalResetVariant=Disabled  TRSumVariant=Passthrough  SumFdbkVariant=Disabled  SumVariant=Sum_PI  TsampFilterVariant=InternalTs  TsampNgainVariant=Passthrough  TsampIntegralVariant=Disabled_SignalSpec  ExternalSaturationOutDataTypeStr=Inherit: Same as second input  DerivativeSourceVariant=Disabled  PreIntVariant=InternalPreInt
  Sum : Sum  Inputs=|+-
  Sum2 : Sum  Inputs=|+-
  Sum{4..7} (4 alike) : Sum  Inputs=|++
  feedforward : Gain  Gain=F
  wCf : Gain  Gain=2*pi*50*Cf
  Idref : Outport
  Iqref : Outport  Port=2
  wires:
  Sum4/1 -> Idref/1
  Sum/1 -> PID Controller/1
  Sum5/1 -> Sum4/1
  feedforward/1 -> Sum6/2
  Sum7/1 -> Sum6/1
  IqL/1 -> feedforward/1
  Vd/1 -> Sum/2, wCf/1
  Vq/1 -> Sum2/2
  PID Controller2/1 -> Sum7/1
  Sum6/1 -> Iqref/1
  Feedforward/1 -> Sum4/2
  wCf/1 -> Sum7/2
  Sum2/1 -> PID Controller2/1
  -wCf/1 -> Sum5/2
  Vdref/1 -> Sum/1
  PID Controller/1 -> Sum5/1
  Vqref/1 -> -wCf/1, Sum2/1
  IdL/1 -> Feedforward/1

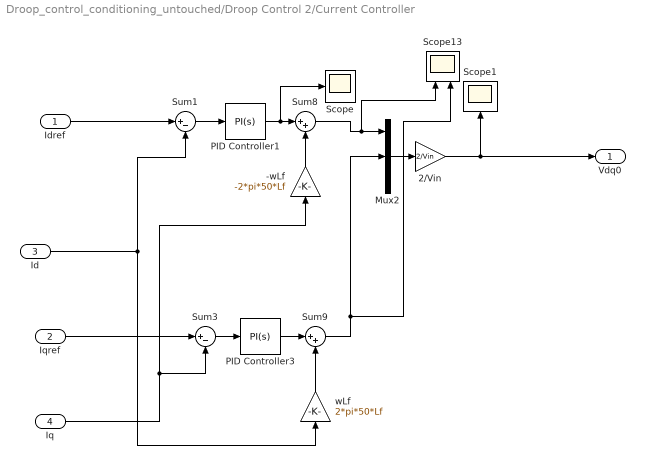
== system Droop_control_conditioning_untouched/Droop Control 2/Current Controller ==
  Idref : Inport
  Iqref : Inport  Port=2
  Id : Inport  Port=3
  Iq : Inport  Port=4
  -wLf : Gain  Gain=-2*pi*50*Lf
  2/Vin : Gain  Gain=2/Vin
  Mux2 : Mux  Inputs=3
  PID Controller1 : slpidlib/PID Controller  Controller=PI  Form=Parallel  TimeDomain=Continuous-time  UseExternalTs=off  SampleTime=Tsample  IntegratorMethod=Forward Euler  FilterMethod=Forward Euler  ControllerParametersSource=internal  P=kpi  I=kii  UseKiTs=off  D=0  UseExternalDerivativeSource=off  N=100  UseFilter=on  TunerSelectOption=Transfer Function Based (PID Tuner App)  InitialConditionSource=internal  InitialConditionForIntegrator=0  InitialConditionForFilter=0  DifferentiatorICPrevScaledInput=0  ExternalReset=none  TrackingMode=off  Kt=1  LimitOutput=off  SatLimitsSource=internal  UpperSaturationLimit=Ilim1  LowerSaturationLimit=Ilim2  LinearizeAsGain=on  AntiWindupMode=none  Kb=1  LimitIntegrator=off  UpperIntegratorSaturationLimit=inf  LowerIntegratorSaturationLimit=-inf  POutMin=[]  POutMax=[]  IOutMin=[]  IOutMax=[]  DOutMin=[]  DOutMax=[]  NOutMin=[]  NOutMax=[]  SumOutMin=[]  SumOutMax=[]  SaturationOutMin=[]  SaturationOutMax=[]  PParamMin=[]  PParamMax=[]  IParamMin=[]  IParamMax=[]  DParamMin=[]  DParamMax=[]  NParamMin=[]  NParamMax=[]  KbParamMin=[]  KbParamMax=[]  KtParamMin=[]  KtParamMax=[]  KbOutMin=[]  KbOutMax=[]  KtOutMin=[]  KtOutMax=[]  IntegratorOutMin=[]  IntegratorOutMax=[]  FilterOutMin=[]  FilterOutMax=[]  SumI1OutMin=[]  SumI1OutMax=[]  SumI2OutMin=[]  SumI2OutMax=[]  SumI3OutMin=[]  SumI3OutMax=[]  SumI4OutMin=[]  SumI4OutMax=[]  SumDOutMin=[]  SumDOutMax=[]  DifferentiatorOutMin=[]  DifferentiatorOutMax=[]  FilterDiffOutCoefMin=[]  FilterDiffOutCoefMax=[]  ReciprocalOutMin=[]  ReciprocalOutMax=[]  SumDenOutMin=[]  SumDenOutMax=[]  SumNumOutMin=[]  SumNumOutMax=[]  DivideOutMin=[]  DivideOutMax=[]  UdiffTsProdOutMin=[]  UdiffTsProdOutMax=[]  NTsProdOutMin=[]  NTsProdOutMax=[]  UintegralTsProdOutMin=[]  UintegralTsProdOutMax=[]  UngainTsProdOutMin=[]  UngainTsProdOutMax=[]  ClampingZeroOutDataTypeStr=Inherit: Inherit via back propagation  ClampingZeroOutMin=[]  ClampingZeroOutMax=[]  FilterDenConstantOutDataTypeStr=Inherit: Inherit via back propagation  FilterDenConstantOutMin=[]  FilterDenConstantOutMax=[]  PCopyOutDataTypeStr=Inherit: Inherit via back propagation  PCopyOutMin=[]  PCopyOutMax=[]  NCopyOutDataTypeStr=Inherit: Inherit via back propagation  NCopyOutMin=[]  NCopyOutMax=[]  IntegratorContinuousStateAttributes=''  IntegratorStateMustResolveToSignalObject=off  IntegratorRTWStateStorageClass=Auto  FilterContinuousStateAttributes=''  FilterStateMustResolveToSignalObject=off  FilterRTWStateStorageClass=Auto  ParallelPVariant=InternalParameters  IdealPVariant=Disabled  IVariant=InternalParameters  DVariant=Disabled  IntegratorVariant=Continuous  SatVariant=Disabled  AWVariant=Passthrough  PCopyVariant=Disabled  TRVariant=Disabled  FdbkBlocksVariant=Forward  IdealPFdbkVariant=Disabled  SatFdbkVariant=Disabled  DerivativeFilterVariant=Disabled  NVariant=Disabled  NCopyVariant=Disabled_SignalSpec  FilterICVariant=Disabled  IntegratorICVariant=InternalICs  ExternalResetVariant=Disabled  TRSumVariant=Passthrough  SumFdbkVariant=Disabled  SumVariant=Sum_PI  TsampFilterVariant=InternalTs  TsampNgainVariant=Passthrough  TsampIntegralVariant=Disabled_SignalSpec  ExternalSaturationOutDataTypeStr=Inherit: Same as second input  DerivativeSourceVariant=Disabled  PreIntVariant=InternalPreInt
  PID Controller3 : slpidlib/PID Controller  Controller=PI  Form=Parallel  TimeDomain=Continuous-time  UseExternalTs=off  SampleTime=Tsample  IntegratorMethod=Forward Euler  FilterMethod=Forward Euler  ControllerParametersSource=internal  P=kpi  I=kii  UseKiTs=off  D=0  UseExternalDerivativeSource=off  N=100  UseFilter=on  TunerSelectOption=Transfer Function Based (PID Tuner App)  InitialConditionSource=internal  InitialConditionForIntegrator=0  InitialConditionForFilter=0  DifferentiatorICPrevScaledInput=0  ExternalReset=none  TrackingMode=off  Kt=1  LimitOutput=off  SatLimitsSource=internal  UpperSaturationLimit=Ilim1  LowerSaturationLimit=Ilim2  LinearizeAsGain=on  AntiWindupMode=none  Kb=1  LimitIntegrator=off  UpperIntegratorSaturationLimit=inf  LowerIntegratorSaturationLimit=-inf  POutMin=[]  POutMax=[]  IOutMin=[]  IOutMax=[]  DOutMin=[]  DOutMax=[]  NOutMin=[]  NOutMax=[]  SumOutMin=[]  SumOutMax=[]  SaturationOutMin=[]  SaturationOutMax=[]  PParamMin=[]  PParamMax=[]  IParamMin=[]  IParamMax=[]  DParamMin=[]  DParamMax=[]  NParamMin=[]  NParamMax=[]  KbParamMin=[]  KbParamMax=[]  KtParamMin=[]  KtParamMax=[]  KbOutMin=[]  KbOutMax=[]  KtOutMin=[]  KtOutMax=[]  IntegratorOutMin=[]  IntegratorOutMax=[]  FilterOutMin=[]  FilterOutMax=[]  SumI1OutMin=[]  SumI1OutMax=[]  SumI2OutMin=[]  SumI2OutMax=[]  SumI3OutMin=[]  SumI3OutMax=[]  SumI4OutMin=[]  SumI4OutMax=[]  SumDOutMin=[]  SumDOutMax=[]  DifferentiatorOutMin=[]  DifferentiatorOutMax=[]  FilterDiffOutCoefMin=[]  FilterDiffOutCoefMax=[]  ReciprocalOutMin=[]  ReciprocalOutMax=[]  SumDenOutMin=[]  SumDenOutMax=[]  SumNumOutMin=[]  SumNumOutMax=[]  DivideOutMin=[]  DivideOutMax=[]  UdiffTsProdOutMin=[]  UdiffTsProdOutMax=[]  NTsProdOutMin=[]  NTsProdOutMax=[]  UintegralTsProdOutMin=[]  UintegralTsProdOutMax=[]  UngainTsProdOutMin=[]  UngainTsProdOutMax=[]  ClampingZeroOutDataTypeStr=Inherit: Inherit via back propagation  ClampingZeroOutMin=[]  ClampingZeroOutMax=[]  FilterDenConstantOutDataTypeStr=Inherit: Inherit via back propagation  FilterDenConstantOutMin=[]  FilterDenConstantOutMax=[]  PCopyOutDataTypeStr=Inherit: Inherit via back propagation  PCopyOutMin=[]  PCopyOutMax=[]  NCopyOutDataTypeStr=Inherit: Inherit via back propagation  NCopyOutMin=[]  NCopyOutMax=[]  IntegratorContinuousStateAttributes=''  IntegratorStateMustResolveToSignalObject=off  IntegratorRTWStateStorageClass=Auto  FilterContinuousStateAttributes=''  FilterStateMustResolveToSignalObject=off  FilterRTWStateStorageClass=Auto  ParallelPVariant=InternalParameters  IdealPVariant=Disabled  IVariant=InternalParameters  DVariant=Disabled  IntegratorVariant=Continuous  SatVariant=Disabled  AWVariant=Passthrough  PCopyVariant=Disabled  TRVariant=Disabled  FdbkBlocksVariant=Forward  IdealPFdbkVariant=Disabled  SatFdbkVariant=Disabled  DerivativeFilterVariant=Disabled  NVariant=Disabled  NCopyVariant=Disabled_SignalSpec  FilterICVariant=Disabled  IntegratorICVariant=InternalICs  ExternalResetVariant=Disabled  TRSumVariant=Passthrough  SumFdbkVariant=Disabled  SumVariant=Sum_PI  TsampFilterVariant=InternalTs  TsampNgainVariant=Passthrough  TsampIntegralVariant=Disabled_SignalSpec  ExternalSaturationOutDataTypeStr=Inherit: Same as second input  DerivativeSourceVariant=Disabled  PreIntVariant=InternalPreInt
  Scope : Scope
  Scope1 : Scope
  Scope13 : Scope  NumInputPorts=2
  Sum1 : Sum  Inputs=|+-
  Sum3 : Sum  Inputs=|+-
  Sum8 : Sum  Inputs=|++
  Sum9 : Sum  Inputs=|++
  wLf : Gain  Gain=2*pi*50*Lf
  Vdq0 : Outport
  wires:
  Iqref/1 -> Sum3/1
  -wLf/1 -> Sum8/2
  Idref/1 -> Sum1/1
  Mux2/1 -> 2/Vin/1
  PID Controller1/1 -> Sum8/1, Scope/1
  Sum3/1 -> PID Controller3/1
  Sum8/1 -> Mux2/1, Scope13/1
  PID Controller3/1 -> Sum9/1
  Sum1/1 -> PID Controller1/1
  Iq/1 -> Sum3/2, -wLf/1
  Id/1 -> wLf/1, Sum1/2
  2/Vin/1 -> Scope1/1, Vdq0/1
  wLf/1 -> Sum9/2
  Sum9/1 -> Mux2/2, Scope13/2

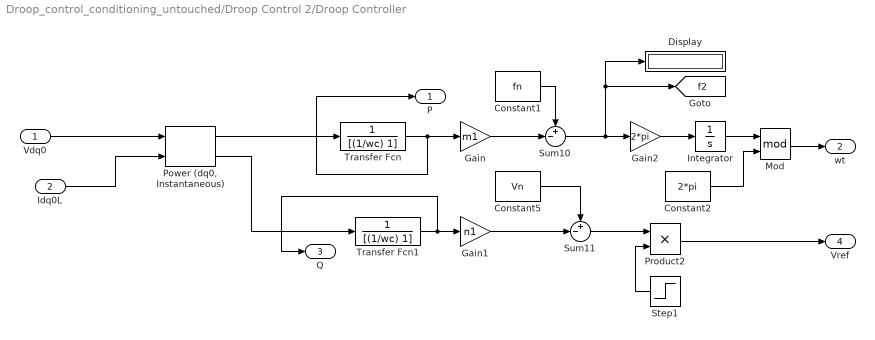
== system Droop_control_conditioning_untouched/Droop Control 2/Droop Controller ==
  Vdq0 : Inport
  Idq0L : Inport  Port=2
  Constant1 : Constant  Value=fn
  Constant2 : Constant  Value=2*pi
  Constant5 : Constant  Value=Vn
  Display : Display
  Gain : Gain  Gain=m1
  Gain1 : Gain  Gain=n1
  Gain2 : Gain  Gain=2*pi
  Integrator : Integrator
  Mod : Math  Operator=mod
  "Power (dq0, Instantaneous)" : spsPowerdq0InstantaneousLib/Power (dq0, Instantaneous)
      settings: LibrarySourceBlock=|
      | sps_lib/Sensors and Measurements/Power
      | (dq0, Instantaneous)
  Product2 : Product  Inputs=**
  Step1 : Step  Time=ts  SampleTime=0
  Sum10 : Sum  Inputs=+-|
  Sum11 : Sum  Inputs=+-|
  Transfer Fcn : TransferFcn  Numerator=[0 1]  Denominator=[(1/wc) 1]
  Transfer Fcn1 : TransferFcn  Numerator=[0 1]  Denominator=[(1/wc) 1]
  P : Outport
  wt : Outport  Port=2
  Q : Outport  Port=3
  Vref : Outport  Port=4
  tag scope: f2=global
  wires:
  Sum11/1 -> Product2/1
  Product2/1 -> Vref/1
  Step1/1 -> Product2/2
  Sum10/1 -> Display/1, [f2], Gain2/1
  Gain2/1 -> Integrator/1
  Idq0L/1 -> "Power (dq0, Instantaneous)"/2
  Vdq0/1 -> "Power (dq0, Instantaneous)"/1
  Constant2/1 -> Mod/2
  Mod/1 -> wt/1
  Integrator/1 -> Mod/1
  Transfer Fcn1/1 -> Gain1/1, Q/1
  Transfer Fcn/1 -> Gain/1, P/1
  Gain/1 -> Sum10/2
  Gain1/1 -> Sum11/2
  Constant5/1 -> Sum11/1
  Constant1/1 -> Sum10/1
  "Power (dq0, Instantaneous)"/1 -> Transfer Fcn/1
  "Power (dq0, Instantaneous)"/2 -> Transfer Fcn1/1

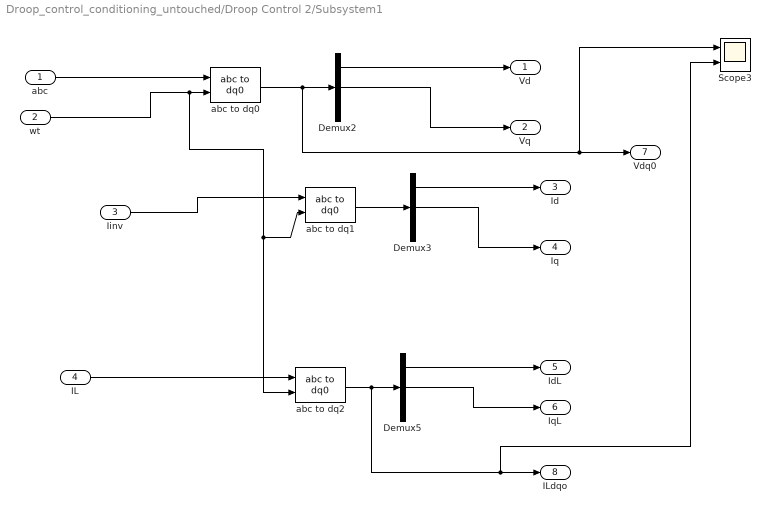
== system Droop_control_conditioning_untouched/Droop Control 2/Subsystem1 ==
  abc : Inport
  wt : Inport  Port=2
  Iinv : Inport  Port=3
  IL : Inport  Port=4
  Demux2 : Demux  Outputs=3
  Demux3 : Demux  Outputs=3
  Demux5 : Demux  Outputs=3
  Scope3 : Scope  NumInputPorts=2
  abc to dq0 : spsabctodq0Lib/abc to dq0  Alignment=90 degrees behind phase A axis
  abc to dq1 : spsabctodq0Lib/abc to dq0  Alignment=90 degrees behind phase A axis
  abc to dq2 : spsabctodq0Lib/abc to dq0  Alignment=90 degrees behind phase A axis
  Vd : Outport
  Vq : Outport  Port=2
  Id : Outport  Port=3
  Iq : Outport  Port=4
  IdL : Outport  Port=5
  IqL : Outport  Port=6
  Vdq0 : Outport  Port=7
  ILdqo : Outport  Port=8
  wires:
  IL/1 -> abc to dq2/1
  Demux3/2 -> Iq/1
  abc/1 -> abc to dq0/1
  Demux5/2 -> IqL/1
  Demux5/1 -> IdL/1
  Demux2/1 -> Vd/1
  Demux3/1 -> Id/1
  Iinv/1 -> abc to dq1/1
  Demux2/2 -> Vq/1
  wt/1 -> abc to dq0/2, abc to dq1/2, abc to dq2/2
  abc to dq1/1 -> Demux3/1
  abc to dq2/1 -> Demux5/1, ILdqo/1, Scope3/2
  abc to dq0/1 -> Demux2/1, Vdq0/1, Scope3/1
